simulink model "Copter_System"  (Simulink 7.4)
settings: Solver=ode4  StartTime=0.0  StopTime=tend  FixedStep=Ts  RelTol=1e-3
values from neighbouring files (symbols this model uses):
  f1 = (I_y-I_z)/I_x    [quadrocopter_param.m]
  f2 = rot.J_z/I_x    [quadrocopter_param.m]
  f3 = (I_z-I_x)/I_y    [quadrocopter_param.m]
  f4 = rot.J_z/I_y    [quadrocopter_param.m]
  f5 = (I_x-I_y)/I_z    [quadrocopter_param.m]
  g = 9.81    [complementary_filter_param.m]    (also in quadrocopter_param.m)
  HPF = 0.95    [complementary_filter_param.m]    (also in quadrocopter_param.m)
  I_x = elec.I_x+bat.I_x+2*boom.I_1x+2*boom.I_1y+2*mot.I_1x+2*mot.I_1y+                             2*rot.I_1x+2*rot.I_1y    [quadrocopter_param.m]
  I_y = elec.I_y+bat.I_y+2*boom.I_1x+2*boom.I_1y+2*mot.I_1x+2*mot.I_1y+                             2*rot.I_1x+2*rot.I_1y    [quadrocopter_param.m]
  I_z = elec.I_z+bat.I_z+4*boom.I_1z+4*mot.I_1z+4*rot.I_1z    [quadrocopter_param.m]
  LPF = 0.05    [complementary_filter_param.m]    (also in quadrocopter_param.m)
  m = elec.m+bat.m+boom.m+(4*mot.m)+(4*rot.m)    [quadrocopter_param.m]
  speed = rpm.*(2*pi/60)    [quadrocopter_param.m]
  thrust = [0.58 1 1.33 2 2.54 3.33 4.08 4.54]    [quadrocopter_param.m]
  Ts = 0.01    [complementary_filter_param.m]    (also in quadrocopter_param.m)
undefined symbols (not defined in the file or in its folder): boom, DiscIntNeverNeededParam
libraries: simulink x7, dspinverses x1
settings Model: Creator=Joachim  LastModifiedBy=Sreekanth
settings DataIOCC: LimitDataPoints=off  SaveOutput=off  SaveState=on
settings DebuggingCC: AlgebraicLoopMsg=none

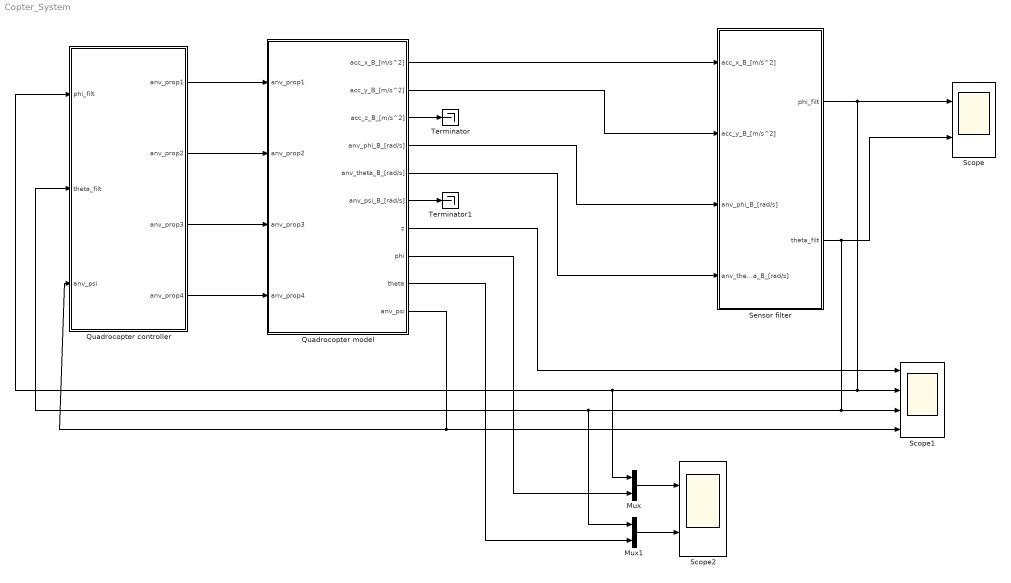
== system Copter_System ==
  Mux : Mux  Inputs=2
  Mux1 : Mux  Inputs=2
  Quadrocopter controller : Subsystem
  Quadrocopter model : Subsystem
  Scope : Scope  NumInputPorts=2
      settings: YMin=-5~-5  YMax=5~5  SaveName=ScopeData12
  Scope1 : Scope  NumInputPorts=4
      settings: YMin=-5~-5~-5~-5  YMax=5~5~5~5  SaveName=ScopeData14
  Scope2 : Scope  NumInputPorts=2
      settings: TimeRange=2.768662838392125  YMin=-0.00272445~-0.0178576  YMax=0.0152582~0.00343767  SaveName=ScopeData15
  Sensor filter : Subsystem
  Terminator : Terminator
  Terminator1 : Terminator
  wires:
  Quadrocopter controller/1(anv_prop1) -> Quadrocopter model/1(anv_prop1)
  Quadrocopter controller/2(anv_prop2) -> Quadrocopter model/2(anv_prop2)
  Quadrocopter controller/3(anv_prop3) -> Quadrocopter model/3(anv_prop3)
  Quadrocopter controller/4(anv_prop4) -> Quadrocopter model/4(anv_prop4)
  Sensor filter/1(phi_filt) -> Scope/1, Scope1/2, Mux/1, Quadrocopter controller/1(phi_filt)
  Sensor filter/2(theta_filt) -> Scope/2, Scope1/3, Mux1/1, Quadrocopter controller/2(theta_filt)
  Mux/1 -> Scope2/1
  Mux1/1 -> Scope2/2
  Quadrocopter model/1(acc_x_B_[m/s^2]) -> Sensor filter/1(acc_x_B_[m/s^2])
  Quadrocopter model/2(acc_y_B_[m/s^2]) -> Sensor filter/2(acc_y_B_[m/s^2])
  Quadrocopter model/3(acc_z_B_[m/s^2]) -> Terminator/1
  Quadrocopter model/6(anv_psi_B_[rad/s]) -> Terminator1/1
  Quadrocopter model/4(anv_phi_B_[rad/s]) -> Sensor filter/3(anv_phi_B_[rad/s])
  Quadrocopter model/5(anv_theta_B_[rad/s]) -> Sensor filter/4(anv_theta_B_[rad/s])
  Quadrocopter model/7(z) -> Scope1/1
  Quadrocopter model/8(phi) -> Mux/2
  Quadrocopter model/9(theta) -> Mux1/2
  Quadrocopter model/10(anv_psi) -> Scope1/4, Quadrocopter controller/3(anv_psi)

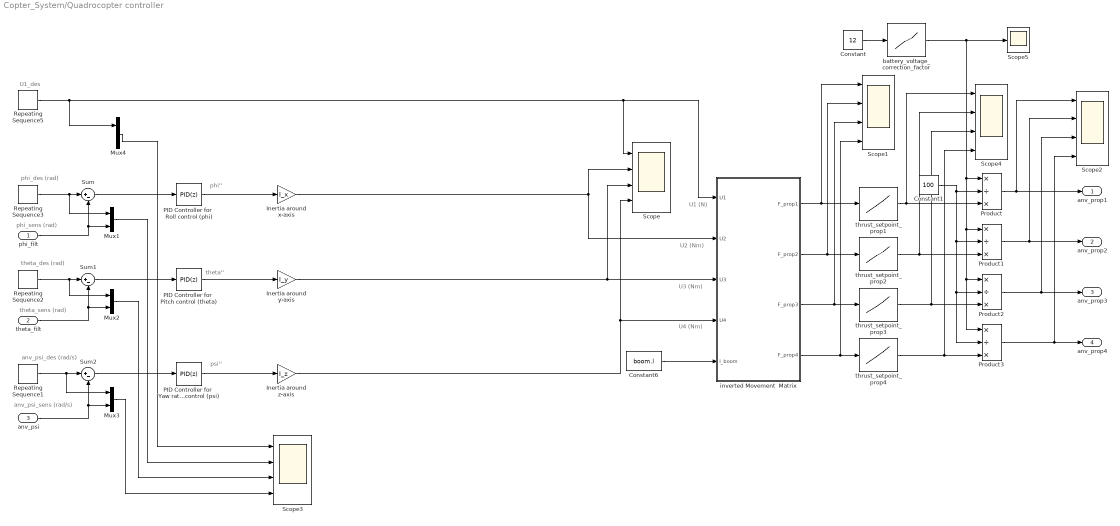
== system Copter_System/Quadrocopter controller ==
  note: U1 (N)
  note: U4 (Nm)
  note: U3 (Nm)
  note: U2 (Nm)
  note: anv_psi_sens (rad/s)
  note: anv_psi_des (rad/s)
  note: theta_sens (rad)
  note: theta_des (rad)
  note: phi_sens (rad)
  note: phi_des (rad)
  note: phi''
  note: theta''
  note: psi''
  note: U1_des
  phi_filt : Inport  OutDataType=fixdt(1, 16)  OutScaling=2^0
  theta_filt : Inport  Port=2  OutDataType=fixdt(1, 16)  OutScaling=2^0
  anv_psi : Inport  Port=3  OutDataType=fixdt(1, 16)  OutScaling=2^0
  Constant : Constant  Value=12  OutDataType=fixdt(1, 16)  OutScaling=2^0
  Constant1 : Constant  Value=100  OutDataType=fixdt(1, 16)  OutScaling=2^0
  Constant6 : Constant  Value=boom.l  OutDataType=fixdt(1, 16)  OutScaling=2^0
  Inertia around x-axis : Gain  Gain=I_x  ParameterDataType=fixdt(1, 16)  ParameterScaling=2^0  OutDataType=fixdt(1, 16)  OutScaling=2^0
  Inertia around y-axis : Gain  Gain=I_y  ParameterDataType=fixdt(1, 16)  ParameterScaling=2^0  OutDataType=fixdt(1, 16)  OutScaling=2^0
  Inertia around z-axis : Gain  Gain=I_z  ParameterDataType=fixdt(1, 16)  ParameterScaling=2^0  OutDataType=fixdt(1, 16)  OutScaling=2^0
  Mux{1..4} (4 alike) : Mux  Inputs=2
  PID Controller for  Pitch control (theta) : simulink/Continuous/PID Controller  DialogController=pidpack.PIDConfig.pidDDGCreate  DialogControllerArgs=DataTag0  SystemSampleTime=-1  Controller=PID  TimeDomain=Discrete-time  SampleTime=Ts  IntegratorMethod=Forward Euler  FilterMethod=Forward Euler  Form=Parallel  P=24.5741408339408  I=2.22368348800941  D=63.7702410156948  N=116.694973399311  InitialConditionSource=internal  InitialConditionForIntegrator=0  InitialConditionForFilter=0  ExternalReset=none  LimitOutput=off  UpperSaturationLimit=20  LowerSaturationLimit=-20  LinearizeAsGain=off  AntiWindupMode=clamping  Kb=1  TrackingMode=off  Kt=1  PParamMin=[]  PParamMax=[]  IParamMin=[]  IParamMax=[]  DParamMin=[]  DParamMax=[]  NParamMin=[]  NParamMax=[]  KbParamMin=[]  KbParamMax=[]  KtParamMin=[]  KtParamMax=[]  POutMin=[]  POutMax=[]  IOutMin=[]  IOutMax=[]  DOutMin=[]  DOutMax=[]  NOutMin=[]  NOutMax=[]  KbOutMin=[]  KbOutMax=[]  KtOutMin=[]  KtOutMax=[]  IntegratorOutMin=[]  IntegratorOutMax=[]  FilterOutMin=[]  FilterOutMax=[]  SumOutMin=[]  SumOutMax=[]  SumI1OutMin=[]  SumI1OutMax=[]  SumI2OutMin=[]  SumI2OutMax=[]  SumI3OutMin=[]  SumI3OutMax=[]  SumDOutMin=[]  SumDOutMax=[]  SaturationOutMin=[]  SaturationOutMax=[]  IntegratorContinuousStateAttributes=''  IntegratorStateMustResolveToSignalObject=off  IntegratorRTWStateStorageClass=Auto  FilterContinuousStateAttributes=''  FilterStateMustResolveToSignalObject=off  FilterRTWStateStorageClass=Auto
  PID Controller for  Roll control (phi) : simulink/Continuous/PID Controller  DialogController=pidpack.PIDConfig.pidDDGCreate  DialogControllerArgs=DataTag1  SystemSampleTime=-1  Controller=PID  TimeDomain=Discrete-time  SampleTime=Ts  IntegratorMethod=Forward Euler  FilterMethod=Forward Euler  Form=Parallel  P=24.7618031261535  I=2.24747518128395  D=64.0360013621  N=116.729970424548  InitialConditionSource=internal  InitialConditionForIntegrator=0  InitialConditionForFilter=0  ExternalReset=none  LimitOutput=off  UpperSaturationLimit=20  LowerSaturationLimit=-20  LinearizeAsGain=off  AntiWindupMode=clamping  Kb=1  TrackingMode=off  Kt=1  PParamMin=[]  PParamMax=[]  IParamMin=[]  IParamMax=[]  DParamMin=[]  DParamMax=[]  NParamMin=[]  NParamMax=[]  KbParamMin=[]  KbParamMax=[]  KtParamMin=[]  KtParamMax=[]  POutMin=[]  POutMax=[]  IOutMin=[]  IOutMax=[]  DOutMin=[]  DOutMax=[]  NOutMin=[]  NOutMax=[]  KbOutMin=[]  KbOutMax=[]  KtOutMin=[]  KtOutMax=[]  IntegratorOutMin=[]  IntegratorOutMax=[]  FilterOutMin=[]  FilterOutMax=[]  SumOutMin=[]  SumOutMax=[]  SumI1OutMin=[]  SumI1OutMax=[]  SumI2OutMin=[]  SumI2OutMax=[]  SumI3OutMin=[]  SumI3OutMax=[]  SumDOutMin=[]  SumDOutMax=[]  SaturationOutMin=[]  SaturationOutMax=[]  IntegratorContinuousStateAttributes=''  IntegratorStateMustResolveToSignalObject=off  IntegratorRTWStateStorageClass=Auto  FilterContinuousStateAttributes=''  FilterStateMustResolveToSignalObject=off  FilterRTWStateStorageClass=Auto
  PID Controller for  Yaw rate control (psi) : simulink/Continuous/PID Controller  DialogController=pidpack.PIDConfig.pidDDGCreate  DialogControllerArgs=DataTag2  SystemSampleTime=-1  Controller=PID  TimeDomain=Discrete-time  SampleTime=Ts  IntegratorMethod=Forward Euler  FilterMethod=Forward Euler  Form=Parallel  P=43.2936626596122  I=27.8858530381629  D=7.7780350767139  N=130.140476991467  InitialConditionSource=internal  InitialConditionForIntegrator=0  InitialConditionForFilter=0  ExternalReset=none  LimitOutput=off  UpperSaturationLimit=180  LowerSaturationLimit=-180  LinearizeAsGain=off  AntiWindupMode=clamping  Kb=1  TrackingMode=off  Kt=1  PParamMin=[]  PParamMax=[]  IParamMin=[]  IParamMax=[]  DParamMin=[]  DParamMax=[]  NParamMin=[]  NParamMax=[]  KbParamMin=[]  KbParamMax=[]  KtParamMin=[]  KtParamMax=[]  POutMin=[]  POutMax=[]  IOutMin=[]  IOutMax=[]  DOutMin=[]  DOutMax=[]  NOutMin=[]  NOutMax=[]  KbOutMin=[]  KbOutMax=[]  KtOutMin=[]  KtOutMax=[]  IntegratorOutMin=[]  IntegratorOutMax=[]  FilterOutMin=[]  FilterOutMax=[]  SumOutMin=[]  SumOutMax=[]  SumI1OutMin=[]  SumI1OutMax=[]  SumI2OutMin=[]  SumI2OutMax=[]  SumI3OutMin=[]  SumI3OutMax=[]  SumDOutMin=[]  SumDOutMax=[]  SaturationOutMin=[]  SaturationOutMax=[]  IntegratorContinuousStateAttributes=''  IntegratorStateMustResolveToSignalObject=off  IntegratorRTWStateStorageClass=Auto  FilterContinuousStateAttributes=''  FilterStateMustResolveToSignalObject=off  FilterRTWStateStorageClass=Auto
  Product{,1..3} (4 alike) : Product  Inputs=*/*  OutDataType=fixdt(1, 16)  OutScaling=2^0  RndMeth=Zero
  Repeating Sequence1 : simulink/Sources/Repeating Sequence  SystemSampleTime=-1  rep_seq_t=desyaw.time  rep_seq_y=desyaw.velocity
  Repeating Sequence2 : simulink/Sources/Repeating Sequence  SystemSampleTime=-1  rep_seq_t=despitch.time  rep_seq_y=despitch.angle
  Repeating Sequence3 : simulink/Sources/Repeating Sequence  SystemSampleTime=-1  rep_seq_t=desroll.time  rep_seq_y=desroll.angle
  Repeating Sequence5 : simulink/Sources/Repeating Sequence  SystemSampleTime=-1  rep_seq_t=desforce.time  rep_seq_y=desforce.force
  Scope{,1..4} (5 alike) : Scope  NumInputPorts=4
      Scope settings: TimeRange=30  YMin=16.5147~0.359533~-0.366931~-0.234953  YMax=16.5153~0.397379~0.366932~0.259685
      Scope1 settings: TimeRange=30  YMin=-5~-5~-5~-5  YMax=5~5~5~5
      Scope2 settings: TimeRange=10  YMin=0~0~0~0  YMax=500~500~500~500  SaveName=ScopeData2
      Scope3 settings: TimeRange=10  YMin=-1e-015~0.359533~0.366931~0.234953  YMax=1e-015~0.397379~0.366932~0.259685  SaveName=ScopeData13
      Scope4 settings: TimeRange=10  YMin=0~0~0~0  YMax=500~500~500~500  SaveName=ScopeData25
  Scope5 : Scope
      settings: TimeRange=10  YMin=0  YMax=150  SaveName=ScopeData26
  Sum : Sum  Inputs=|+-  OutDataType=fixdt(1, 16)  OutScaling=2^0
  Sum1 : Sum  Inputs=|+-  OutDataType=fixdt(1, 16)  OutScaling=2^0
  Sum2 : Sum  Inputs=|+-  OutDataType=fixdt(1, 16)  OutScaling=2^0
  battery_voltage_correction_factor : Lookup  InputValues=[10 12]  Table=[120 100]  LookUpMeth=Interpolation-Use End Values  OutDataType=fixdt(1, 16)  OutScaling=2^0
  inverted Movement  Matrix : Stateflow chart
  thrust_setpoint_prop{1..4} (4 alike) : Lookup  InputValues=[0 500 4500]./1000  Table=[0 40 175]  LookUpMeth=Interpolation-Use End Values  OutDataType=fixdt(1, 16)  OutScaling=2^0
  anv_prop1 : Outport  OutDataType=fixdt(1, 16)  OutScaling=2^0
  anv_prop2 : Outport  Port=2  OutDataType=fixdt(1, 16)  OutScaling=2^0
  anv_prop3 : Outport  Port=3  OutDataType=fixdt(1, 16)  OutScaling=2^0
  anv_prop4 : Outport  Port=4  OutDataType=fixdt(1, 16)  OutScaling=2^0
  wires:
  Repeating Sequence1/1 -> Sum2/1, Mux3/1
  Repeating Sequence2/1 -> Sum1/1, Mux2/1
  Repeating Sequence3/1 -> Sum/1, Mux1/1
  theta_filt/1 -> Sum1/2, Mux2/2
  anv_psi/1 -> Sum2/2, Mux3/2
  phi_filt/1 -> Sum/2, Mux1/2
  inverted Movement  Matrix/4(F_prop4) -> Scope1/4, thrust_setpoint_prop4/1
  inverted Movement  Matrix/3(F_prop3) -> Scope1/3, thrust_setpoint_prop3/1
  inverted Movement  Matrix/2(F_prop2) -> Scope1/2, thrust_setpoint_prop2/1
  inverted Movement  Matrix/1(F_prop1) -> Scope1/1, thrust_setpoint_prop1/1
  Inertia around x-axis/1 -> inverted Movement  Matrix/2(U2), Scope/2
  Constant6/1 -> inverted Movement  Matrix/5(l_boom)
  Inertia around z-axis/1 -> inverted Movement  Matrix/4(U4), Scope/4
  Inertia around y-axis/1 -> inverted Movement  Matrix/3(U3), Scope/3
  PID Controller for  Yaw rate control (psi)/1 -> Inertia around z-axis/1
  PID Controller for  Pitch control (theta)/1 -> Inertia around y-axis/1
  PID Controller for  Roll control (phi)/1 -> Inertia around x-axis/1
  Sum2/1 -> PID Controller for  Yaw rate control (psi)/1
  Sum1/1 -> PID Controller for  Pitch control (theta)/1
  Sum/1 -> PID Controller for  Roll control (phi)/1
  Mux1/1 -> Scope3/2
  Mux2/1 -> Scope3/3
  Mux3/1 -> Scope3/4
  Repeating Sequence5/1 -> Mux4/1, Scope/1, inverted Movement  Matrix/1(U1)
  Mux4/1 -> Scope3/1
  Constant/1 -> battery_voltage_correction_factor/1
  thrust_setpoint_prop1/1 -> Product/3, Scope4/1
  Constant1/1 -> Product/2, Product1/2, Product2/2, Product3/2
  Product/1 -> anv_prop1/1, Scope2/1
  thrust_setpoint_prop4/1 -> Product3/3, Scope4/4
  thrust_setpoint_prop3/1 -> Product2/3, Scope4/3
  thrust_setpoint_prop2/1 -> Product1/3, Scope4/2
  Product1/1 -> anv_prop2/1, Scope2/2
  Product2/1 -> anv_prop3/1, Scope2/3
  Product3/1 -> anv_prop4/1, Scope2/4
  battery_voltage_correction_factor/1 -> Product3/1, Product2/1, Product1/1, Product/1, Scope5/1

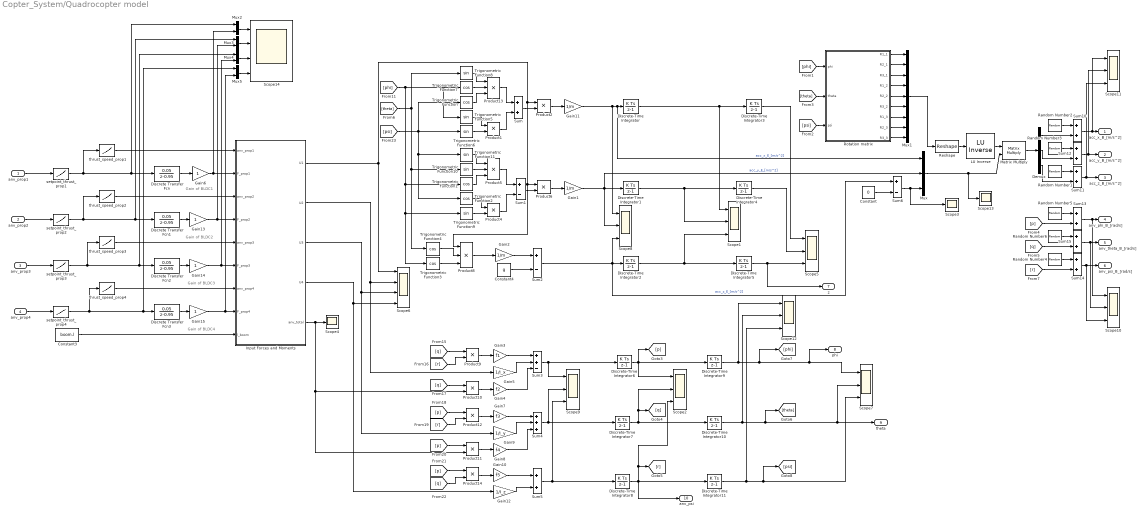
== system Copter_System/Quadrocopter model ==
  note: Gain of BLDC1
  note: Gain of BLDC2
  note: Gain of BLDC3
  note: Gain of BLDC4
  anv_prop1 : Inport  OutDataType=fixdt(1, 16)  OutScaling=2^0
  anv_prop2 : Inport  Port=2  OutDataType=fixdt(1, 16)  OutScaling=2^0
  anv_prop3 : Inport  Port=3  OutDataType=fixdt(1, 16)  OutScaling=2^0
  anv_prop4 : Inport  Port=4  OutDataType=fixdt(1, 16)  OutScaling=2^0
  " LU Inverse" : dspinverses/ LU Inverse  SystemSampleTime=-1
  Constant : Constant  Value=0  OutDataType=fixdt(1, 16)  OutScaling=2^0  SampleTime=Ts
  Constant3 : Constant  Value=boom.l  OutDataType=fixdt(1, 16)  OutScaling=2^0
  Constant4 : Constant  Value=g  OutDataType=fixdt(1, 16)  OutScaling=2^0  SampleTime=Ts
  Demux : Demux  Outputs=3
  Discrete Transfer Fcn{,1..3} (4 alike) : DiscreteTransferFcn  Numerator=[0.05]  Denominator=[1 -0.95]  SampleTime=Ts
  Discrete-Time Integrator{,1..11} (12 alike) : DiscreteIntegrator  SampleTime=Ts  OutDataType=fixdt(1, 16)  OutScaling=2^0  ICPrevOutput=DiscIntNeverNeededParam  ICPrevScaledInput=DiscIntNeverNeededParam
  Gain1 : Gain  Gain=1/m  ParameterDataType=fixdt(1, 16)  ParameterScaling=2^0  OutDataType=fixdt(1, 16)  OutScaling=2^0
  Gain10 : Gain  Gain=f5  ParameterDataType=fixdt(1, 16)  ParameterScaling=2^0  OutDataType=fixdt(1, 16)  OutScaling=2^0
  Gain11 : Gain  Gain=1/m  ParameterDataType=fixdt(1, 16)  ParameterScaling=2^0  OutDataType=fixdt(1, 16)  OutScaling=2^0
  Gain12 : Gain  Gain=1/I_z  ParameterDataType=fixdt(1, 16)  ParameterScaling=2^0  OutDataType=fixdt(1, 16)  OutScaling=2^0
  Gain{6,13..15} (4 alike) : Gain  ParameterDataType=fixdt(1, 16)  ParameterScaling=2^0  OutDataType=fixdt(1, 16)  OutScaling=2^0
  Gain2 : Gain  Gain=1/m  ParameterDataType=fixdt(1, 16)  ParameterScaling=2^0  OutDataType=fixdt(1, 16)  OutScaling=2^0
  Gain3 : Gain  Gain=f1  ParameterDataType=fixdt(1, 16)  ParameterScaling=2^0  OutDataType=fixdt(1, 16)  OutScaling=2^0
  Gain4 : Gain  Gain=f2  ParameterDataType=fixdt(1, 16)  ParameterScaling=2^0  OutDataType=fixdt(1, 16)  OutScaling=2^0
  Gain5 : Gain  Gain=1/I_x  ParameterDataType=fixdt(1, 16)  ParameterScaling=2^0  OutDataType=fixdt(1, 16)  OutScaling=2^0
  Gain7 : Gain  Gain=f3  ParameterDataType=fixdt(1, 16)  ParameterScaling=2^0  OutDataType=fixdt(1, 16)  OutScaling=2^0
  Gain8 : Gain  Gain=f4  ParameterDataType=fixdt(1, 16)  ParameterScaling=2^0  OutDataType=fixdt(1, 16)  OutScaling=2^0
  Gain9 : Gain  Gain=1/I_y  ParameterDataType=fixdt(1, 16)  ParameterScaling=2^0  OutDataType=fixdt(1, 16)  OutScaling=2^0
  Input Forces and Moments : Stateflow chart
  Matrix Multiply : Product  Multiplication=Matrix(*)  OutDataType=sfix(16)  OutScaling=2^0
  Mux : Mux  Inputs=3
  Mux1 : Mux  Inputs=9
  Mux{2..5} (4 alike) : Mux  Inputs=2
  Product{1..2,4,6,9..12,14} (9 alike) : Product  OutDataType=fixdt(1, 16)  OutScaling=2^0  RndMeth=Zero
  Product13 : Product  Inputs=3  OutDataType=fixdt(1, 16)  OutScaling=2^0  RndMeth=Zero
  Product5 : Product  Inputs=3  OutDataType=fixdt(1, 16)  OutScaling=2^0  RndMeth=Zero
  Product8 : Product  Inputs=3  OutDataType=fixdt(1, 16)  OutScaling=2^0  RndMeth=Zero
  Random Number{1..6} (6 alike) : RandomNumber  Variance=0  SampleTime=Ts
  Reshape : Reshape  OutputDimensionality=Customize  OutputDimensions=[3,3]
  Rotation matrix : Stateflow chart
  Scope{1..2,5,7..12} (9 alike) : Scope  NumInputPorts=3
      Scope1 settings: YMin=-5~-5~-5  YMax=5~5~5  SaveName=ScopeData21
      Scope10 settings: YMin=-5~-5~-5  YMax=5~5~5  SaveName=ScopeData9
      Scope11 settings: YMin=-5~-5~-5  YMax=5~5~5  SaveName=ScopeData10
      Scope12 settings: YMin=-5~-5~-5  YMax=5~5~5  SaveName=ScopeData11
      Scope2 settings: YMin=-5~-5~-5  YMax=5~5~5  SaveName=ScopeData24
      Scope5 settings: YMin=-5~-5~-5  YMax=5~5~5  SaveName=ScopeData3
      Scope7 settings: TimeRange=30  YMin=-0.05~-0.2~-0.5  YMax=0.3~0.15~3  SaveName=ScopeData6
      Scope8 settings: TimeRange=30  YMin=-1~-1~3  YMax=1~1~10  SaveName=ScopeData7
      Scope9 settings: YMin=-5~-5~-5  YMax=5~5~5  SaveName=ScopeData8
  Scope13 : Scope
      settings: SaveName=ScopeData22
  Scope14 : Scope  NumInputPorts=4
      settings: YMin=-5~-5~-5~-5  YMax=5~5~5~5  SaveName=ScopeData23
  Scope3 : Scope
      settings: SaveName=ScopeData19
  Scope4 : Scope
      settings: SaveName=ScopeData4
  Scope6 : Scope  NumInputPorts=4
      settings: YMin=-5~-5~-5~-5  YMax=5~5~5~5  SaveName=ScopeData5
  Sum{,5,10..15} (8 alike) : Sum  OutDataType=fixdt(1, 16)  OutScaling=2^0
  Sum1 : Sum  Inputs=+-  OutDataType=fixdt(1, 16)  OutScaling=2^0
  Sum2 : Sum  Inputs=+-  OutDataType=fixdt(1, 16)  OutScaling=2^0
  Sum3 : Sum  Inputs=++-  OutDataType=fixdt(1, 16)  OutScaling=2^0
  Sum4 : Sum  Inputs=+++  OutDataType=fixdt(1, 16)  OutScaling=2^0
  Sum6 : Sum  Inputs=+-  OutDataType=fixdt(1, 16)  OutScaling=2^0
  Trigonometric Function{,1..4,7} (6 alike) : Trigonometry  Operator=cos
  Trigonometric Function{5..6,8..11} (6 alike) : Trigonometry
  setpoint_thrust_prop{1..4} (4 alike) : Lookup  InputValues=[0 40 175]  Table=[0 500 4500]./1000  LookUpMeth=Interpolation-Use End Values  OutDataType=fixdt(1, 16)  OutScaling=2^0
  thrust_speed_prop{1..4} (4 alike) : Lookup  InputValues=thrust  Table=speed  LookUpMeth=Interpolation-Use End Values  OutDataType=fixdt(1, 16)  OutScaling=2^0
  acc_x_B_[m/s^2] : Outport  OutDataType=fixdt(1, 16)  OutScaling=2^0
  acc_y_B_[m/s^2] : Outport  Port=2  OutDataType=fixdt(1, 16)  OutScaling=2^0
  acc_z_B_[m/s^2] : Outport  Port=3  OutDataType=fixdt(1, 16)  OutScaling=2^0
  anv_phi_B_[rad/s] : Outport  Port=4  OutDataType=fixdt(1, 16)  OutScaling=2^0
  anv_theta_B_[rad/s] : Outport  Port=5  OutDataType=fixdt(1, 16)  OutScaling=2^0
  anv_psi_B_[rad/s] : Outport  Port=6  OutDataType=fixdt(1, 16)  OutScaling=2^0
  z : Outport  Port=7  OutDataType=fixdt(1, 16)  OutScaling=2^0
  phi : Outport  Port=8  OutDataType=fixdt(1, 16)  OutScaling=2^0
  theta : Outport  Port=9  OutDataType=fixdt(1, 16)  OutScaling=2^0
  anv_psi : Outport  Port=10  OutDataType=fixdt(1, 16)  OutScaling=2^0
  wires:
  Sum14/1 -> Scope10/3, anv_psi_B_[rad/s]/1
  Sum15/1 -> Scope10/2, anv_theta_B_[rad/s]/1
  Sum13/1 -> Scope10/1, anv_phi_B_[rad/s]/1
  [q] -> Sum15/2
  Random Number6/1 -> Sum15/1
  [r] -> Sum14/2
  Random Number4/1 -> Sum14/1
  [p] -> Sum13/2
  Random Number5/1 -> Sum13/1
  Sum11/1 -> Scope11/3, acc_z_B_[m/s^2]/1
  Sum12/1 -> Scope11/2, acc_y_B_[m/s^2]/1
  Sum10/1 -> Scope11/1, acc_x_B_[m/s^2]/1
  Demux/2 -> Sum12/2
  Random Number3/1 -> Sum12/1
  Demux/3 -> Sum11/2
  Random Number1/1 -> Sum11/1
  Demux/1 -> Sum10/2
  Random Number2/1 -> Sum10/1
  Matrix Multiply/1 -> Demux/1
  anv_prop3/1 -> setpoint_thrust_prop3/1
  anv_prop4/1 -> setpoint_thrust_prop4/1
  Reshape/1 -> " LU Inverse"/1
  Mux/1 -> Matrix Multiply/2, Scope13/1
  Mux1/1 -> Reshape/1
  Rotation matrix/9(R3_3) -> Mux1/9
  Rotation matrix/8(R2_3) -> Mux1/8
  Rotation matrix/7(R1_3) -> Mux1/7
  Rotation matrix/6(R3_2) -> Mux1/6
  Rotation matrix/5(R2_2) -> Mux1/5
  Rotation matrix/4(R1_2) -> Mux1/4
  Rotation matrix/3(R3_1) -> Mux1/3
  Rotation matrix/2(R2_1) -> Mux1/2
  Rotation matrix/1(R1_1) -> Mux1/1
  [psi] -> Rotation matrix/3(psi)
  [theta] -> Rotation matrix/2(theta)
  [phi] -> Rotation matrix/1(phi)
  anv_prop2/1 -> setpoint_thrust_prop2/1
  anv_prop1/1 -> setpoint_thrust_prop1/1
  Constant4/1 -> Sum2/2
  Trigonometric Function4/1 -> Product8/2
  Trigonometric Function3/1 -> Product8/3
  Gain2/1 -> Sum2/1
  Gain11/1 -> Scope8/1, Discrete-Time Integrator/1, Mux/1  "acc_x_E_[m/s^2]"
  Product6/1 -> Gain1/1
  Sum1/1 -> Product6/2
  Product5/1 -> Sum1/1
  Trigonometric Function1/1 -> Product5/3
  Trigonometric Function10/1 -> Product5/2
  Trigonometric Function11/1 -> Product5/1
  Product4/1 -> Sum1/2
  Trigonometric Function2/1 -> Product4/1
  Trigonometric Function9/1 -> Product4/2
  Product2/1 -> Gain11/1
  Sum/1 -> Product2/2
  Product13/1 -> Sum/1
  Trigonometric Function/1 -> Product13/3
  Trigonometric Function7/1 -> Product13/2
  Trigonometric Function8/1 -> Product13/1
  Product1/1 -> Sum/2
  Trigonometric Function5/1 -> Product1/1
  Trigonometric Function6/1 -> Product1/2
  [psi] -> Trigonometric Function2/1, Trigonometric Function11/1, Trigonometric Function/1, Trigonometric Function6/1
  Discrete-Time Integrator/1 -> Scope1/1, Discrete-Time Integrator3/1
  Discrete-Time Integrator1/1 -> Scope1/2, Discrete-Time Integrator4/1
  Discrete-Time Integrator2/1 -> Scope1/3, Discrete-Time Integrator5/1
  [theta] -> Trigonometric Function10/1, Trigonometric Function4/1, Trigonometric Function8/1
  Gain1/1 -> Scope8/2, Discrete-Time Integrator1/1, Mux/2  "acc_y_E_[m/s^2]"
  [phi] -> Trigonometric Function9/1, Trigonometric Function3/1, Trigonometric Function1/1, Trigonometric Function7/1, Trigonometric Function5/1
  Product8/1 -> Gain2/1
  Sum2/1 -> Scope8/3, Discrete-Time Integrator2/1, Sum6/1  "acc_z_E_[m/s^2]"
  Discrete-Time Integrator3/1 -> Scope5/1
  Discrete-Time Integrator4/1 -> Scope5/2
  Discrete-Time Integrator5/1 -> Scope5/3, z/1
  Constant3/1 -> Input Forces and Moments/9(l_boom)
  Sum5/1 -> Scope9/3, Discrete-Time Integrator8/1
  Input Forces and Moments/4(U4) -> Scope6/4, Gain12/1
  Gain12/1 -> Sum5/2
  Gain10/1 -> Sum5/1
  Product14/1 -> Gain10/1
  [q] -> Product14/2
  [p] -> Product14/1
  Sum4/1 -> Scope9/2, Discrete-Time Integrator7/1
  Input Forces and Moments/3(U3) -> Scope6/3, Gain9/1
  Gain8/1 -> Sum4/3
  Gain9/1 -> Sum4/2
  Product11/1 -> Gain8/1
  [p] -> Product11/1
  Gain7/1 -> Sum4/1
  Product12/1 -> Gain7/1
  [r] -> Product12/2
  [p] -> Product12/1
  Input Forces and Moments/1(U1) -> Product8/1, Product6/1, Product2/1, Scope6/1
  Sum3/1 -> Scope9/1, Discrete-Time Integrator6/1
  Gain4/1 -> Sum3/3
  Gain5/1 -> Sum3/2
  Input Forces and Moments/2(U2) -> Scope6/2, Gain5/1
  Product10/1 -> Gain4/1
  [q] -> Product10/1
  Gain3/1 -> Sum3/1
  Product9/1 -> Gain3/1
  [r] -> Product9/2
  [q] -> Product9/1
  Input Forces and Moments/5(anv_total) -> Product11/2, Product10/2, Scope4/1
  Discrete-Time Integrator9/1 -> Scope12/1, [phi], Scope7/1, phi/1
  Discrete-Time Integrator10/1 -> Scope12/2, [theta], Scope7/2, theta/1
  Discrete-Time Integrator11/1 -> Scope12/3, Scope7/3, [psi]
  Discrete-Time Integrator6/1 -> Scope2/1, [p], Discrete-Time Integrator9/1
  Discrete-Time Integrator7/1 -> Scope2/2, [q], Discrete-Time Integrator10/1
  Discrete-Time Integrator8/1 -> Scope2/3, [r], anv_psi/1, Discrete-Time Integrator11/1
  Constant/1 -> Sum6/2
  Sum6/1 -> Mux/3, Scope3/1
  " LU Inverse"/1 -> Matrix Multiply/1
  Discrete Transfer Fcn/1 -> Gain6/1
  Discrete Transfer Fcn1/1 -> Gain13/1
  Discrete Transfer Fcn2/1 -> Gain14/1
  Discrete Transfer Fcn3/1 -> Gain15/1
  Mux2/1 -> Scope14/1
  Gain6/1 -> Input Forces and Moments/2(F_prop1), Mux2/2
  Gain13/1 -> Input Forces and Moments/4(F_prop2), Mux3/2
  Gain14/1 -> Input Forces and Moments/6(F_prop3), Mux4/2
  Gain15/1 -> Input Forces and Moments/8(F_prop4), Mux5/2
  Mux3/1 -> Scope14/2
  Mux4/1 -> Scope14/3
  Mux5/1 -> Scope14/4
  thrust_speed_prop1/1 -> Input Forces and Moments/1(anv_prop1)
  thrust_speed_prop3/1 -> Input Forces and Moments/5(anv_prop3)
  thrust_speed_prop4/1 -> Input Forces and Moments/7(anv_prop4)
  thrust_speed_prop2/1 -> Input Forces and Moments/3(anv_prop2)
  setpoint_thrust_prop1/1 -> thrust_speed_prop1/1, Mux2/1, Discrete Transfer Fcn/1
  setpoint_thrust_prop2/1 -> thrust_speed_prop2/1, Discrete Transfer Fcn1/1, Mux3/1
  setpoint_thrust_prop3/1 -> thrust_speed_prop3/1, Discrete Transfer Fcn2/1, Mux4/1
  setpoint_thrust_prop4/1 -> thrust_speed_prop4/1, Discrete Transfer Fcn3/1, Mux5/1

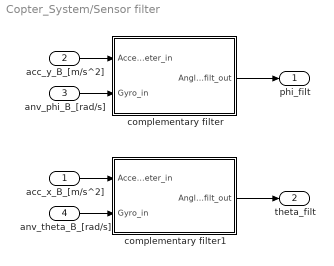
== system Copter_System/Sensor filter ==
  acc_x_B_[m/s^2] : Inport
  acc_y_B_[m/s^2] : Inport  Port=2
  anv_phi_B_[rad/s] : Inport  Port=3
  anv_theta_B_[rad/s] : Inport  Port=4
  complementary filter : Subsystem
  complementary filter1 : Subsystem
  phi_filt : Outport
  theta_filt : Outport  Port=2
  wires:
  complementary filter/1(Angle_filt_out) -> phi_filt/1
  anv_phi_B_[rad/s]/1 -> complementary filter/2(Gyro_in)
  complementary filter1/1(Angle_filt_out) -> theta_filt/1
  anv_theta_B_[rad/s]/1 -> complementary filter1/2(Gyro_in)
  acc_x_B_[m/s^2]/1 -> complementary filter1/1(Accelerometer_in)
  acc_y_B_[m/s^2]/1 -> complementary filter/1(Accelerometer_in)

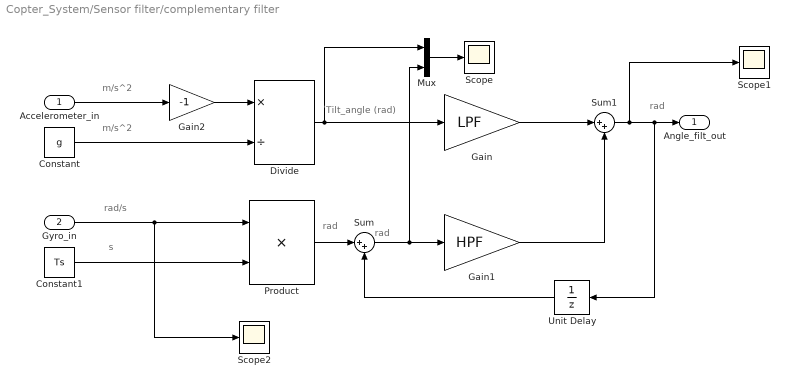
== system Copter_System/Sensor filter/complementary filter ==
  note: rad
  note: rad
  note: rad
  note: s
  note: rad/s
  note: m/s^2
  note: m/s^2
  note: Tilt_angle (rad)
  Accelerometer_in : Inport  OutDataType=fixdt(1, 16)  OutScaling=2^0
  Gyro_in : Inport  Port=2  OutDataType=fixdt(1, 16)  OutScaling=2^0
  Constant : Constant  Value=g  OutDataType=fixdt(1, 16)  OutScaling=2^0  SampleTime=Ts
  Constant1 : Constant  Value=Ts  OutDataType=fixdt(1, 16)  OutScaling=2^0  SampleTime=Ts
  Divide : Product  Inputs=*/  OutDataType=fixdt(1, 16)  OutScaling=2^-10
  Gain : Gain  Gain=LPF  ParameterDataType=fixdt(1, 16)  ParameterScaling=2^0  OutDataType=fixdt(1, 16)  OutScaling=2^0
  Gain1 : Gain  Gain=HPF  ParameterDataType=fixdt(1, 16)  ParameterScaling=2^0  OutDataType=fixdt(1, 16)  OutScaling=2^0
  Gain2 : Gain  Gain=-1  ParameterDataType=fixdt(1, 16)  ParameterScaling=2^0  OutDataType=fixdt(1, 16)  OutScaling=2^0
  Mux : Mux  Inputs=2
  Product : Product  OutDataType=fixdt(1, 16)  OutScaling=2^0  RndMeth=Zero
  Scope : Scope
      settings: SaveName=ScopeData16
  Scope1 : Scope
      settings: SaveName=ScopeData17
  Scope2 : Scope
      settings: SaveName=ScopeData20
  Sum : Sum  Inputs=|++  OutDataType=fixdt(1, 16)  OutScaling=2^0
  Sum1 : Sum  Inputs=|++  OutDataType=fixdt(1, 16)  OutScaling=2^0
  Unit Delay : UnitDelay  SampleTime=-1
  Angle_filt_out : Outport  OutDataType=fixdt(1, 16)  OutScaling=2^0
  wires:
  Constant/1 -> Divide/2
  Accelerometer_in/1 -> Gain2/1
  Gyro_in/1 -> Product/1, Scope2/1
  Constant1/1 -> Product/2
  Sum/1 -> Gain1/1, Mux/2
  Sum1/1 -> Angle_filt_out/1, Unit Delay/1, Scope1/1
  Gain1/1 -> Sum1/2
  Gain/1 -> Sum1/1
  Product/1 -> Sum/1
  Divide/1 -> Gain/1, Mux/1
  Mux/1 -> Scope/1
  Unit Delay/1 -> Sum/2
  Gain2/1 -> Divide/1

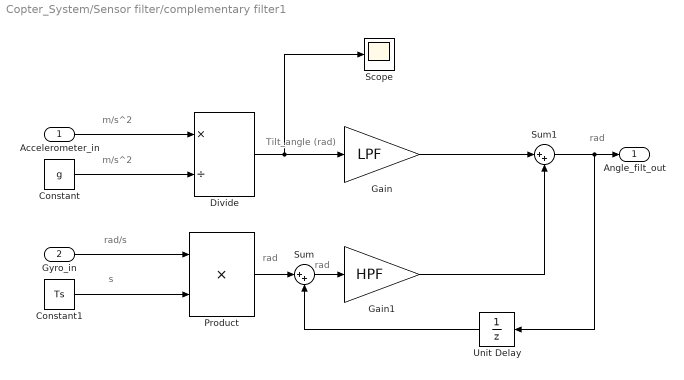
== system Copter_System/Sensor filter/complementary filter1 ==
  note: Tilt_angle (rad)
  note: m/s^2
  note: m/s^2
  note: rad/s
  note: s
  note: rad
  note: rad
  note: rad
  Accelerometer_in : Inport  OutDataType=fixdt(1, 16)  OutScaling=2^0
  Gyro_in : Inport  Port=2  OutDataType=fixdt(1, 16)  OutScaling=2^0
  Constant : Constant  Value=g  OutDataType=fixdt(1, 16)  OutScaling=2^0  SampleTime=Ts
  Constant1 : Constant  Value=Ts  OutDataType=fixdt(1, 16)  OutScaling=2^0  SampleTime=Ts
  Divide : Product  Inputs=*/  OutDataType=fixdt(1, 16)  OutScaling=2^-10
  Gain : Gain  Gain=LPF  ParameterDataType=fixdt(1, 16)  ParameterScaling=2^0  OutDataType=fixdt(1, 16)  OutScaling=2^0
  Gain1 : Gain  Gain=HPF  ParameterDataType=fixdt(1, 16)  ParameterScaling=2^0  OutDataType=fixdt(1, 16)  OutScaling=2^0
  Product : Product  OutDataType=fixdt(1, 16)  OutScaling=2^0  RndMeth=Zero
  Scope : Scope
      settings: SaveName=ScopeData18
  Sum : Sum  Inputs=|++  OutDataType=fixdt(1, 16)  OutScaling=2^0
  Sum1 : Sum  Inputs=|++  OutDataType=fixdt(1, 16)  OutScaling=2^0
  Unit Delay : UnitDelay  SampleTime=-1
  Angle_filt_out : Outport  OutDataType=fixdt(1, 16)  OutScaling=2^0
  wires:
  Divide/1 -> Gain/1, Scope/1
  Product/1 -> Sum/1
  Gain/1 -> Sum1/1
  Gain1/1 -> Sum1/2
  Sum1/1 -> Angle_filt_out/1, Unit Delay/1
  Sum/1 -> Gain1/1
  Constant1/1 -> Product/2
  Gyro_in/1 -> Product/1
  Accelerometer_in/1 -> Divide/1
  Constant/1 -> Divide/2
  Unit Delay/1 -> Sum/2

== matlab function Quadrocopter model/Input Forces and Moments ==
  data: anv_prop1 input double; F_prop1 input double; anv_prop2 input double; F_prop2 input double; anv_prop3 input double; F_prop3 input double; anv_prop4 input double; U1 output double; F_prop4 input double; U2 output double; U3 output double; U4 output double; l_boom input double; anv_total output double
function [U1, U2, U3, U4, anv_total] = input(anv_prop1,F_prop1,anv_prop2,...
    F_prop2,anv_prop3,F_prop3,anv_prop4,F_prop4,l_boom)
%#eml

% Calculating Thrust in z-axis with respect to body fixed coordinate system
U1 = F_prop1 + F_prop2 + F_prop3 + F_prop4;             % [N]

% Calculating Torque around x-axis (Roll) due to Thrust
U2 = l_boom*(-F_prop4+F_prop2);                         % [Nm]

% Calculating Torque around y-axis (Pitch) due to Thrust
U3 = l_boom*(-F_prop1+F_prop3);                         % [Nm]

% Calculating Torque around z-axis (Yaw) due to Thrust
U4 = l_boom*(F_prop1-F_prop2+F_prop3-F_prop4);          % [Nm]

% Overall propeller speed
anv_total = anv_prop1-anv_prop2+anv_prop3-anv_prop4;    % [rad/s]

== matlab function Quadrocopter controller/inverted Movement Matrix ==
  data: U1 input double; F_prop1 output double; F_prop2 output double; F_prop3 output double; F_prop4 output double; U2 input double; U3 input double; U4 input double; l_boom input double
function [F_prop1,F_prop2,F_prop3,F_prop4] = fcn(U1,U2,U3,U4,l_boom)
%#eml

% Force needed at the front propeller in [N]
F_prop1 = (U1/4)-(U3/(2*l_boom))+(U4/(4*l_boom));

% Force needed at the left propeller in [N]
F_prop2 = (U1/4)+(U2/(2*l_boom))-(U4/(4*l_boom));

% Force needed at the back propeller in [N]
F_prop3 = (U1/4)+(U3/(2*l_boom))+(U4/(4*l_boom));

% Force needed at the right propeller in [N]
F_prop4 = (U1/4)-(U2/(2*l_boom))-(U4/(4*l_boom));

== matlab function Quadrocopter model/Rotation matrix ==
  data: phi input double; theta input double; psi input double; R1_1 output double; R2_1 output double; R3_1 output double; R1_2 output double; R2_2 output double; R3_2 output double; R1_3 output double; R2_3 output double; R3_3 output double
function [ R1_1, R2_1, R3_1, R1_2, R2_2, R3_2, R1_3, R2_3, R3_3] = input...
                                                    (phi, theta, psi)
% Transformation of E-frame to B-Frame
R1_1 = cos(psi)*cos(theta);
R2_1 = sin(psi)*cos(theta);
R3_1 = -sin(theta);
R1_2 = -sin(psi)*cos(phi)+cos(psi)*sin(theta)*sin(phi);
R2_2 = cos(psi)*cos(phi)+sin(psi)*sin(theta)*sin(phi);
R3_2 = cos(theta)*sin(phi);
R1_3 = sin(psi)*sin(phi)+cos(psi)*sin(theta)*cos(phi);
R2_3 = -cos(psi)*sin(phi)+sin(psi)*sin(theta)*cos(phi);
R3_3 = cos(theta)*cos(phi);
